simulink model "EV_Modeling_old"  (R2024b)
settings: Solver=FixedStepAuto  StartTime=0.0  StopTime=10382  FixedStep=0.1  RelTol=1e-3
values from neighbouring files (symbols this model uses):
  battery_SOC_SOC = battery_SOC(:,1)    [EV_Truck.m]    (also in simulink.m)
  battery_SOC_voltage = battery_SOC(:,2)    [EV_Truck.m]    (also in simulink.m)
  drag_coefficient_FV1 = table2array(drag_coefficient(:,3))    [simulink.m]
  drag_coefficient_FV2 = table2array(drag_coefficient(:,4))    [simulink.m]
  drag_coefficient_input = table2array(drag_coefficient(:,1))    [simulink.m]
  drag_coefficient_LV = table2array(drag_coefficient(:,2))    [simulink.m]
  electric_consumption_ressistancce = electric_consumption(:,2)    [EV_Truck.m]    (also in simulink.m)
  electric_consumption_voltage = electric_consumption(:,1)    [EV_Truck.m]    (also in simulink.m)
  motor_efficiency_efficiency = table2array(motor_efficiency(2:height(motor_efficiency),2:width(motor_efficiency)))    [EV_Truck.m]    (also in simulink.m)
  motor_efficiency_RPM = table2array(motor_efficiency(2:height(motor_efficiency),1))    [EV_Truck.m]    (also in simulink.m)
  motor_efficiency_torque = transpose(motor_efficiency_torque)    [EV_Truck.m]    (also in simulink.m)
  motor_RPM_torque = table2array(motor_torque(1:14,1))    [EV_Truck.m]    (also in simulink.m)
  motor_torque_RPM = table2array(motor_torque(1:14,2))    [EV_Truck.m]    (also in simulink.m)
undefined symbols (not defined in the file or in its folder): battery_builder_rtmsupport, battery_sli_rtmsupport, C1_mat, C2_mat, c_sqrt, DiscIntNeverNeededParam, dV0_mat, gcbh, n, Wc, Wm, x0
libraries: simulink x87, packLibrary_lib x30, nesl_utility x6, fl_lib x6, simulink_extras x3, mpcadaslib x2, slpidlib x1
(part 12 of 12)

== system EV_Modeling_old/FV2/SOC Estimator (Kalman Filter)1/Kalman Filter/UKBF 2RC/Prediction-correction/Xdot/Sigma points derivatives ==
  A : Inport
  Fi : Inport  Port=2
  x1 : Inport  Port=3
  Assignment : Assignment  NumberOfDimensions=2  DiagnosticForDimensions=Warning  IndexOptions=Index vector (dialog),Index vector (dialog)  Indices=1:n,1  OutputSizes=1,1
  Assignment1 : Assignment  NumberOfDimensions=2  DiagnosticForDimensions=Warning  IndexOptions=Index vector (dialog),Index vector (dialog)  Indices=1:n,2:n+1  OutputSizes=1,1
  Assignment2 : Assignment  NumberOfDimensions=2  DiagnosticForDimensions=Warning  IndexOptions=Index vector (dialog),Index vector (dialog)  Indices=1:n,n+2:2*n+1  OutputSizes=1,1
  Constant : Constant  Value=zeros(n,2*n+1)
  Constant1 : Constant  Value=ones(1,n)  VectorParams1D=off
  Gain : Gain  Gain=c_sqrt
  Matrix Multiply : Product  Multiplication=Matrix(*)
  Matrix Multiply1 : Product  Multiplication=Matrix(*)
  Sum : Sum  Inputs=|++
  Sum1 : Sum  Inputs=|+-
  Xdot : Outport
  wires:
  x1/1 -> Matrix Multiply/1, Assignment/2
  Constant1/1 -> Matrix Multiply/2
  Matrix Multiply/1 -> Sum1/1, Sum/1
  Gain/1 -> Sum1/2, Sum/2
  Sum/1 -> Assignment1/2
  Sum1/1 -> Assignment2/2
  Constant/1 -> Assignment/1
  Assignment/1 -> Assignment1/1
  Assignment1/1 -> Assignment2/1
  Assignment2/1 -> Xdot/1
  A/1 -> Matrix Multiply1/1
  Fi/1 -> Matrix Multiply1/2
  Matrix Multiply1/1 -> Gain/1

== system EV_Modeling_old/FV2/SOC Estimator (Kalman Filter)1/Kalman Filter/UKBF 2RC/Prediction-correction/Xdot/Update Fi ==
  A : Inport
  XWf : Inport  Port=2
  fWX : Inport  Port=3
  K : Inport  Port=4
  Constant1 : Constant  Value=double(Q_2RC)
  Constant4 : Constant  Value=eye(size(P0_2RC,1))
  Constant5 : Constant  Value=double(R)
  Divide1 : Product  Inputs=*/  Multiplication=Matrix(*)
  Gain5 : Gain  Gain=tril(ones(n)-diag(0.5*ones(1,n)))
  Matrix Multiply7 : Product  Inputs=3  Multiplication=Matrix(*)
  Matrix Multiply8 : Product  Inputs=3  Multiplication=Matrix(*)
  Sum3 : Sum  Inputs=+++-
  Transpose3 : Math  Operator=transpose
  Transpose4 : Math  Operator=transpose
  Fi : Outport
  wires:
  A/1 -> Divide1/2
  Matrix Multiply7/1 -> Gain5/1  "M"
  Constant1/1 -> Sum3/3
  Sum3/1 -> Matrix Multiply7/2
  Transpose3/1 -> Matrix Multiply8/3
  Matrix Multiply8/1 -> Sum3/4
  Divide1/1 -> Transpose4/1, Matrix Multiply7/1
  K/1 -> Transpose3/1, Matrix Multiply8/1
  XWf/1 -> Sum3/1
  Constant4/1 -> Divide1/1
  Transpose4/1 -> Matrix Multiply7/3
  Constant5/1 -> Matrix Multiply8/2
  fWX/1 -> Sum3/2
  Gain5/1 -> Fi/1  "Fi"

== system EV_Modeling_old/FV2/SOC Estimator (Kalman Filter)1/Kalman Filter/UKF/Prediction/Measurement function/Measurement function ==
  Current : Inport
  Temperature : Inport  Port=2
  x : Inport  Port=3
  Add2 : Sum  Inputs=+--
  Get SOC : Selector  InputPortWidth=2  IndexOptions=Index vector (dialog)  Indices=[1]  OutputSizes=1
  Get V1 : Selector  InputPortWidth=2  IndexOptions=Index vector (dialog)  Indices=2  OutputSizes=1
  OCV Table : Lookup_n-D  BreakpointsForDimension1=SOC_vec  BreakpointsForDimension2=T_vec  BeginIndexSearchUsingPreviousIndexResult=on  Table=V0_mat  ExtrapMethod=Clip  InternalRulePriority=Speed  RndMeth=Simplest
      settings: InputPortMap=u0,u1
  Product2 : Product
  R0 Table : Lookup_n-D  BreakpointsForDimension1=SOC_vec  BreakpointsForDimension2=T_vec  BeginIndexSearchUsingPreviousIndexResult=on  Table=R0_mat  ExtrapMethod=Clip  InternalRulePriority=Speed  RndMeth=Simplest
      settings: InputPortMap=u0,u1
  y : Outport
  wires:
  x/1 -> Get SOC/1, Get V1/1
  OCV Table/1 -> Add2/1
  Current/1 -> Product2/2
  Get SOC/1 -> OCV Table/1, R0 Table/1
  Get V1/1 -> Add2/3  "U1"
  Product2/1 -> Add2/2
  Add2/1 -> y/1
  R0 Table/1 -> Product2/1
  Temperature/1 -> R0 Table/2, OCV Table/2

== system EV_Modeling_old/FV2/SOC Estimator (Kalman Filter)1/Kalman Filter/UKF/Prediction/State function/State function ==
  Current : Inport
  Temperature : Inport  Port=2
  x : Inport  Port=3
  Add : Sum
  Add1 : Sum  Inputs=-+
  C1 : Lookup_n-D  BreakpointsForDimension1=SOC_vec  BreakpointsForDimension2=T_vec  BeginIndexSearchUsingPreviousIndexResult=on  Table=C1_mat  ExtrapMethod=Clip  InternalRulePriority=Speed  RndMeth=Simplest
      settings: InputPortMap=u0,u1
  Divide1 : Product  Inputs=*/
  Divide2 : Product  Inputs=*/
  Gain : Gain  Gain=-1/(AH*3600)
  Get SOC : Selector  InputPortWidth=2  IndexOptions=Index vector (dialog)  Indices=1  OutputSizes=1
  Get V1 : Selector  InputPortWidth=2  IndexOptions=Index vector (dialog)  Indices=2  OutputSizes=1
  Mux : Mux  Inputs=2
  Probe : Probe  ProbeWidth=off  ProbeComplexSignal=off  ProbeSampleTimeDataType=Same as input
  Product : Product  OutDataTypeStr=single
  Product1 : Product
  R1 : Lookup_n-D  BreakpointsForDimension1=SOC_vec  BreakpointsForDimension2=T_vec  BeginIndexSearchUsingPreviousIndexResult=on  Table=R1_mat  ExtrapMethod=Clip  InternalRulePriority=Speed  RndMeth=Simplest
      settings: InputPortMap=u0,u1
  Selector : Selector  InputPortWidth=2  IndexOptions=Index vector (dialog)  Indices=1  OutputSizes=1
  xk1 : Outport
  wires:
  Gain/1 -> Mux/1
  Temperature/1 -> R1/2, C1/2
  x/1 -> Get SOC/1, Get V1/1, Add/1
  Product/1 -> Add/2
  Add1/1 -> Mux/2  "xdot_2"
  Add/1 -> xk1/1
  Divide2/1 -> Add1/1
  Mux/1 -> Product/1  "xdot"
  Selector/1 -> Product/2
  Current/1 -> Probe/1, Divide1/1, Gain/1  "Current"
  C1/1 -> Divide1/2, Product1/2  "C1"
  Get V1/1 -> Divide2/1
  R1/1 -> Product1/1  "R1"
  Get SOC/1 -> R1/1, C1/1
  Product1/1 -> Divide2/2  "R1*C1"
  Divide1/1 -> Add1/2  "Current/C1"
  Probe/1 -> Selector/1

== system EV_Modeling_old/FV2/SOC Estimator (Kalman Filter)1/Kalman Filter/UKF 2RC/Prediction/Measurement function/Measurement function ==
  Current : Inport
  Temperature : Inport  Port=2
  x : Inport  Port=3
  Add2 : Sum  Inputs=+---
  Get SOC : Selector  InputPortWidth=3  IndexOptions=Index vector (dialog)  Indices=[1]  OutputSizes=1
  Get V1 : Selector  InputPortWidth=3  IndexOptions=Index vector (dialog)  Indices=2  OutputSizes=1
  Get V2 : Selector  InputPortWidth=3  IndexOptions=Index vector (dialog)  Indices=3  OutputSizes=1
  OCV Table : Lookup_n-D  BreakpointsForDimension1=SOC_vec  BreakpointsForDimension2=T_vec  BeginIndexSearchUsingPreviousIndexResult=on  Table=V0_mat  ExtrapMethod=Clip  InternalRulePriority=Speed  RndMeth=Simplest
      settings: InputPortMap=u0,u1
  Product2 : Product
  R0 Table : Lookup_n-D  BreakpointsForDimension1=SOC_vec  BreakpointsForDimension2=T_vec  BeginIndexSearchUsingPreviousIndexResult=on  Table=R0_mat  ExtrapMethod=Clip  InternalRulePriority=Speed  RndMeth=Simplest
      settings: InputPortMap=u0,u1
  y : Outport
  wires:
  Get V2/1 -> Add2/4  "V2"
  x/1 -> Get SOC/1, Get V1/1, Get V2/1
  OCV Table/1 -> Add2/1
  Current/1 -> Product2/2
  Get SOC/1 -> OCV Table/1, R0 Table/1
  Get V1/1 -> Add2/3  "V1"
  Product2/1 -> Add2/2
  Add2/1 -> y/1
  R0 Table/1 -> Product2/1
  Temperature/1 -> R0 Table/2, OCV Table/2

== system EV_Modeling_old/FV2/SOC Estimator (Kalman Filter)1/Kalman Filter/UKF 2RC/Prediction/State function/State function ==
  Current : Inport
  Temperature : Inport  Port=2
  x : Inport  Port=3
  Add : Sum
  Add1 : Sum  Inputs=-+
  Add2 : Sum  Inputs=-+
  C1 : Lookup_n-D  BreakpointsForDimension1=SOC_vec  BreakpointsForDimension2=T_vec  BeginIndexSearchUsingPreviousIndexResult=on  Table=C1_mat  ExtrapMethod=Clip  InternalRulePriority=Speed  RndMeth=Simplest
      settings: InputPortMap=u0,u1
  C2 : Lookup_n-D  BreakpointsForDimension1=SOC_vec  BreakpointsForDimension2=T_vec  Table=C2_mat  InternalRulePriority=Speed  RndMeth=Simplest
      settings: InputPortMap=u0,u1
  Divide{1..4} (4 alike) : Product  Inputs=*/
  Gain : Gain  Gain=-1/(AH*3600)
  Get SOC : Selector  InputPortWidth=3  IndexOptions=Index vector (dialog)  Indices=1  OutputSizes=1
  Get V1 : Selector  InputPortWidth=3  IndexOptions=Index vector (dialog)  Indices=2  OutputSizes=1
  Get V2 : Selector  InputPortWidth=3  IndexOptions=Index vector (dialog)  Indices=3  OutputSizes=1
  Mux : Mux  Inputs=3
  Probe : Probe  ProbeWidth=off  ProbeComplexSignal=off  ProbeSampleTimeDataType=Same as input
  Product : Product  OutDataTypeStr=single
  Product1 : Product
  Product2 : Product
  R1 : Lookup_n-D  BreakpointsForDimension1=SOC_vec  BreakpointsForDimension2=T_vec  BeginIndexSearchUsingPreviousIndexResult=on  Table=R1_mat  ExtrapMethod=Clip  InternalRulePriority=Speed  RndMeth=Simplest
      settings: InputPortMap=u0,u1
  R2 : Lookup_n-D  BreakpointsForDimension1=SOC_vec  BreakpointsForDimension2=T_vec  Table=R2_mat  InternalRulePriority=Speed  RndMeth=Simplest
      settings: InputPortMap=u0,u1
  Selector : Selector  InputPortWidth=2  IndexOptions=Index vector (dialog)  Indices=1  OutputSizes=1
  xk1 : Outport
  wires:
  Get V2/1 -> Divide3/1
  Add2/1 -> Mux/3  "xdot_3"
  Divide4/1 -> Add2/2  "Current/C2"
  Divide3/1 -> Add2/1
  Product2/1 -> Divide3/2  "R2*C2"
  C2/1 -> Product2/2, Divide4/2  "C2"
  R2/1 -> Product2/1  "R2"
  Gain/1 -> Mux/1
  Temperature/1 -> R1/2, C1/2, R2/2, C2/2
  x/1 -> Get SOC/1, Get V1/1, Add/1, Get V2/1
  Product/1 -> Add/2
  Add1/1 -> Mux/2  "xdot_2"
  Add/1 -> xk1/1
  Divide2/1 -> Add1/1
  Mux/1 -> Product/1  "xdot"
  Selector/1 -> Product/2
  Current/1 -> Probe/1, Divide1/1, Gain/1, Divide4/1  "Current"
  C1/1 -> Divide1/2, Product1/2  "C1"
  Get V1/1 -> Divide2/1
  R1/1 -> Product1/1  "R1"
  Get SOC/1 -> R1/1, C1/1, R2/1, C2/1
  Product1/1 -> Divide2/2  "R1*C1"
  Divide1/1 -> Add1/2  "Current/C1"
  Probe/1 -> Selector/1

== system EV_Modeling_old/LV/SOC Estimator (Kalman Filter)/Kalman Filter/UKBF/Prediction-correction/Measurement function/Measurement function ==
  Current : Inport
  Temperature : Inport  Port=2
  x : Inport  Port=3
  Add2 : Sum  Inputs=+--
  Get SOC1 : Selector  InputPortWidth=2  IndexOptions=Index vector (dialog)  Indices=[1]  OutputSizes=1
  Get V1 : Selector  InputPortWidth=2  IndexOptions=Index vector (dialog)  Indices=2  OutputSizes=1
  OCV Table : Lookup_n-D  BreakpointsForDimension1=SOC_vec  BreakpointsForDimension2=T_vec  BeginIndexSearchUsingPreviousIndexResult=on  Table=V0_mat  ExtrapMethod=Clip  InternalRulePriority=Speed  RndMeth=Simplest
      settings: InputPortMap=u0,u1
  Product2 : Product
  R0 Table : Lookup_n-D  BreakpointsForDimension1=SOC_vec  BreakpointsForDimension2=T_vec  BeginIndexSearchUsingPreviousIndexResult=on  Table=R0_mat  ExtrapMethod=Clip  InternalRulePriority=Speed  RndMeth=Simplest
      settings: InputPortMap=u0,u1
  y : Outport
  wires:
  x/1 -> Get SOC1/1, Get V1/1
  OCV Table/1 -> Add2/1
  Current/1 -> Product2/2
  Get SOC1/1 -> OCV Table/1, R0 Table/1  "SOC"
  Get V1/1 -> Add2/3
  Product2/1 -> Add2/2
  Add2/1 -> y/1
  R0 Table/1 -> Product2/1
  Temperature/1 -> R0 Table/2, OCV Table/2

== system EV_Modeling_old/LV/SOC Estimator (Kalman Filter)/Kalman Filter/UKBF/Prediction-correction/State function/State function ==
  Current : Inport
  Temperature : Inport  Port=2
  x : Inport  Port=3
  Add1 : Sum  Inputs=-+
  C1 : Lookup_n-D  BreakpointsForDimension1=SOC_vec  BreakpointsForDimension2=T_vec  BeginIndexSearchUsingPreviousIndexResult=on  Table=C1_mat  ExtrapMethod=Clip  InternalRulePriority=Speed  RndMeth=Simplest
      settings: InputPortMap=u0,u1
  Divide1 : Product  Inputs=*/
  Divide2 : Product  Inputs=*/
  Gain : Gain  Gain=-1/(AH*3600)
  Get SOC : Selector  InputPortWidth=2  IndexOptions=Index vector (dialog)  Indices=1  OutputSizes=1
  Get V1 : Selector  InputPortWidth=2  IndexOptions=Index vector (dialog)  Indices=2  OutputSizes=1
  Mux : Mux  Inputs=2
  Product1 : Product
  R1 : Lookup_n-D  BreakpointsForDimension1=SOC_vec  BreakpointsForDimension2=T_vec  BeginIndexSearchUsingPreviousIndexResult=on  Table=R1_mat  ExtrapMethod=Clip  InternalRulePriority=Speed  RndMeth=Simplest
      settings: InputPortMap=u0,u1
  f(x) : Outport
  wires:
  Gain/1 -> Mux/1
  Temperature/1 -> R1/2, C1/2
  x/1 -> Get SOC/1, Get V1/1
  Add1/1 -> Mux/2  "xdot_2"
  Divide2/1 -> Add1/1
  Mux/1 -> f(x)/1  "xdot"
  Current/1 -> Divide1/1, Gain/1  "Current"
  C1/1 -> Divide1/2, Product1/2  "C1"
  Get V1/1 -> Divide2/1  "V1"
  R1/1 -> Product1/1  "R1"
  Get SOC/1 -> R1/1, C1/1
  Product1/1 -> Divide2/2  "R1*C1"
  Divide1/1 -> Add1/2  "Current/C1"

== system EV_Modeling_old/LV/SOC Estimator (Kalman Filter)/Kalman Filter/UKBF/Prediction-correction/Xdot/Sigma points derivatives ==
  A : Inport
  Fi : Inport  Port=2
  x1 : Inport  Port=3
  Assignment : Assignment  NumberOfDimensions=2  DiagnosticForDimensions=Warning  IndexOptions=Index vector (dialog),Index vector (dialog)  Indices=1:n,1  OutputSizes=1,1
  Assignment1 : Assignment  NumberOfDimensions=2  DiagnosticForDimensions=Warning  IndexOptions=Index vector (dialog),Index vector (dialog)  Indices=1:n,2:n+1  OutputSizes=1,1
  Assignment2 : Assignment  NumberOfDimensions=2  DiagnosticForDimensions=Warning  IndexOptions=Index vector (dialog),Index vector (dialog)  Indices=1:n,n+2:2*n+1  OutputSizes=1,1
  Constant : Constant  Value=zeros(n,2*n+1)
  Constant1 : Constant  Value=ones(1,n)  VectorParams1D=off
  Gain : Gain  Gain=c_sqrt
  Matrix Multiply : Product  Multiplication=Matrix(*)
  Matrix Multiply1 : Product  Multiplication=Matrix(*)
  Sum : Sum  Inputs=|++
  Sum1 : Sum  Inputs=|+-
  Xdot : Outport
  wires:
  x1/1 -> Matrix Multiply/1, Assignment/2
  Constant1/1 -> Matrix Multiply/2
  Matrix Multiply/1 -> Sum1/1, Sum/1
  Gain/1 -> Sum1/2, Sum/2
  Sum/1 -> Assignment1/2
  Sum1/1 -> Assignment2/2
  Constant/1 -> Assignment/1
  Assignment/1 -> Assignment1/1
  Assignment1/1 -> Assignment2/1
  Assignment2/1 -> Xdot/1
  A/1 -> Matrix Multiply1/1
  Fi/1 -> Matrix Multiply1/2
  Matrix Multiply1/1 -> Gain/1

== system EV_Modeling_old/LV/SOC Estimator (Kalman Filter)/Kalman Filter/UKBF/Prediction-correction/Xdot/Update Fi ==
  A : Inport
  XWf : Inport  Port=2
  fWX : Inport  Port=3
  K : Inport  Port=4
  Constant1 : Constant  Value=double(Q)
  Constant4 : Constant  Value=eye(size(P0,1))
  Constant5 : Constant  Value=double(R)
  Divide1 : Product  Inputs=*/  Multiplication=Matrix(*)
  Gain5 : Gain  Gain=tril(ones(n)-diag(0.5*ones(1,n)))
  Matrix Multiply7 : Product  Inputs=3  Multiplication=Matrix(*)
  Matrix Multiply8 : Product  Inputs=3  Multiplication=Matrix(*)
  Sum3 : Sum  Inputs=+++-
  Transpose3 : Math  Operator=transpose
  Transpose4 : Math  Operator=transpose
  Fi : Outport
  wires:
  A/1 -> Divide1/2
  Matrix Multiply7/1 -> Gain5/1  "M"
  Constant1/1 -> Sum3/3
  Sum3/1 -> Matrix Multiply7/2
  Transpose3/1 -> Matrix Multiply8/3
  Matrix Multiply8/1 -> Sum3/4
  Divide1/1 -> Transpose4/1, Matrix Multiply7/1
  K/1 -> Transpose3/1, Matrix Multiply8/1
  XWf/1 -> Sum3/1
  Constant4/1 -> Divide1/1
  Transpose4/1 -> Matrix Multiply7/3
  Constant5/1 -> Matrix Multiply8/2
  fWX/1 -> Sum3/2
  Gain5/1 -> Fi/1  "Fi"

== system EV_Modeling_old/LV/SOC Estimator (Kalman Filter)/Kalman Filter/UKBF 2RC/Prediction-correction/Measurement function/Measurement function ==
  Current : Inport
  Temperature : Inport  Port=2
  x : Inport  Port=3
  Add2 : Sum  Inputs=+---
  Get SOC1 : Selector  InputPortWidth=3  IndexOptions=Index vector (dialog)  Indices=[1]  OutputSizes=1
  Get V1 : Selector  InputPortWidth=3  IndexOptions=Index vector (dialog)  Indices=2  OutputSizes=1
  Get V2 : Selector  InputPortWidth=3  IndexOptions=Index vector (dialog)  Indices=3  OutputSizes=1
  OCV Table : Lookup_n-D  BreakpointsForDimension1=SOC_vec  BreakpointsForDimension2=T_vec  BeginIndexSearchUsingPreviousIndexResult=on  Table=V0_mat  ExtrapMethod=Clip  InternalRulePriority=Speed  RndMeth=Simplest
      settings: InputPortMap=u0,u1
  Product2 : Product
  R0 Table : Lookup_n-D  BreakpointsForDimension1=SOC_vec  BreakpointsForDimension2=T_vec  BeginIndexSearchUsingPreviousIndexResult=on  Table=R0_mat  ExtrapMethod=Clip  InternalRulePriority=Speed  RndMeth=Simplest
      settings: InputPortMap=u0,u1
  y : Outport
  wires:
  Get V2/1 -> Add2/4
  x/1 -> Get SOC1/1, Get V1/1, Get V2/1
  OCV Table/1 -> Add2/1
  Current/1 -> Product2/2
  Get SOC1/1 -> OCV Table/1, R0 Table/1  "SOC"
  Get V1/1 -> Add2/3
  Product2/1 -> Add2/2
  Add2/1 -> y/1
  R0 Table/1 -> Product2/1
  Temperature/1 -> R0 Table/2, OCV Table/2

== system EV_Modeling_old/LV/SOC Estimator (Kalman Filter)/Kalman Filter/UKBF 2RC/Prediction-correction/State function/State function ==
  Current : Inport
  Temperature : Inport  Port=2
  x : Inport  Port=3
  2-D Lookup Table C2 : Lookup_n-D  BreakpointsForDimension1=SOC_vec  BreakpointsForDimension2=T_vec  Table=C2_mat  InternalRulePriority=Speed  RndMeth=Simplest
      settings: InputPortMap=u0,u1
  2-D Lookup Table R2 : Lookup_n-D  BreakpointsForDimension1=SOC_vec  BreakpointsForDimension2=T_vec  Table=R2_mat  InternalRulePriority=Speed  RndMeth=Simplest
      settings: InputPortMap=u0,u1
  Add1 : Sum  Inputs=-+
  Add2 : Sum  Inputs=-+
  C1 : Lookup_n-D  BreakpointsForDimension1=SOC_vec  BreakpointsForDimension2=T_vec  BeginIndexSearchUsingPreviousIndexResult=on  Table=C1_mat  ExtrapMethod=Clip  InternalRulePriority=Speed  RndMeth=Simplest
      settings: InputPortMap=u0,u1
  Divide{1..4} (4 alike) : Product  Inputs=*/
  Gain : Gain  Gain=-1/(AH*3600)
  Get SOC : Selector  InputPortWidth=3  IndexOptions=Index vector (dialog)  Indices=1  OutputSizes=1
  Get V1 : Selector  InputPortWidth=3  IndexOptions=Index vector (dialog)  Indices=2  OutputSizes=1
  Get V2 : Selector  InputPortWidth=3  IndexOptions=Index vector (dialog)  Indices=3  OutputSizes=1
  Mux : Mux  Inputs=3
  Product1 : Product
  Product2 : Product
  R1 : Lookup_n-D  BreakpointsForDimension1=SOC_vec  BreakpointsForDimension2=T_vec  BeginIndexSearchUsingPreviousIndexResult=on  Table=R1_mat  ExtrapMethod=Clip  InternalRulePriority=Speed  RndMeth=Simplest
      settings: InputPortMap=u0,u1
  f(x) : Outport
  wires:
  Divide4/1 -> Add2/2  "Current/C2"
  Divide3/1 -> Add2/1
  Add2/1 -> Mux/3  "xdot_3"
  Product2/1 -> Divide3/2  "R1*C1"
  Get V2/1 -> Divide3/1  "V2"
  2-D Lookup Table C2/1 -> Product2/2, Divide4/2  "C2"
  2-D Lookup Table R2/1 -> Product2/1  "R2"
  Gain/1 -> Mux/1
  Temperature/1 -> R1/2, C1/2, 2-D Lookup Table R2/2, 2-D Lookup Table C2/2
  x/1 -> Get SOC/1, Get V1/1, Get V2/1
  Add1/1 -> Mux/2  "xdot_2"
  Divide2/1 -> Add1/1
  Mux/1 -> f(x)/1  "xdot"
  Current/1 -> Divide1/1, Gain/1, Divide4/1  "Current"
  C1/1 -> Divide1/2, Product1/2  "C1"
  Get V1/1 -> Divide2/1  "V1"
  R1/1 -> Product1/1  "R1"
  Get SOC/1 -> R1/1, C1/1, 2-D Lookup Table R2/1, 2-D Lookup Table C2/1
  Product1/1 -> Divide2/2  "R1*C1"
  Divide1/1 -> Add1/2  "Current/C1"

== system EV_Modeling_old/LV/SOC Estimator (Kalman Filter)/Kalman Filter/UKBF 2RC/Prediction-correction/Xdot/Sigma points derivatives ==
  A : Inport
  Fi : Inport  Port=2
  x1 : Inport  Port=3
  Assignment : Assignment  NumberOfDimensions=2  DiagnosticForDimensions=Warning  IndexOptions=Index vector (dialog),Index vector (dialog)  Indices=1:n,1  OutputSizes=1,1
  Assignment1 : Assignment  NumberOfDimensions=2  DiagnosticForDimensions=Warning  IndexOptions=Index vector (dialog),Index vector (dialog)  Indices=1:n,2:n+1  OutputSizes=1,1
  Assignment2 : Assignment  NumberOfDimensions=2  DiagnosticForDimensions=Warning  IndexOptions=Index vector (dialog),Index vector (dialog)  Indices=1:n,n+2:2*n+1  OutputSizes=1,1
  Constant : Constant  Value=zeros(n,2*n+1)
  Constant1 : Constant  Value=ones(1,n)  VectorParams1D=off
  Gain : Gain  Gain=c_sqrt
  Matrix Multiply : Product  Multiplication=Matrix(*)
  Matrix Multiply1 : Product  Multiplication=Matrix(*)
  Sum : Sum  Inputs=|++
  Sum1 : Sum  Inputs=|+-
  Xdot : Outport
  wires:
  x1/1 -> Matrix Multiply/1, Assignment/2
  Constant1/1 -> Matrix Multiply/2
  Matrix Multiply/1 -> Sum1/1, Sum/1
  Gain/1 -> Sum1/2, Sum/2
  Sum/1 -> Assignment1/2
  Sum1/1 -> Assignment2/2
  Constant/1 -> Assignment/1
  Assignment/1 -> Assignment1/1
  Assignment1/1 -> Assignment2/1
  Assignment2/1 -> Xdot/1
  A/1 -> Matrix Multiply1/1
  Fi/1 -> Matrix Multiply1/2
  Matrix Multiply1/1 -> Gain/1

== system EV_Modeling_old/LV/SOC Estimator (Kalman Filter)/Kalman Filter/UKBF 2RC/Prediction-correction/Xdot/Update Fi ==
  A : Inport
  XWf : Inport  Port=2
  fWX : Inport  Port=3
  K : Inport  Port=4
  Constant1 : Constant  Value=double(Q_2RC)
  Constant4 : Constant  Value=eye(size(P0_2RC,1))
  Constant5 : Constant  Value=double(R)
  Divide1 : Product  Inputs=*/  Multiplication=Matrix(*)
  Gain5 : Gain  Gain=tril(ones(n)-diag(0.5*ones(1,n)))
  Matrix Multiply7 : Product  Inputs=3  Multiplication=Matrix(*)
  Matrix Multiply8 : Product  Inputs=3  Multiplication=Matrix(*)
  Sum3 : Sum  Inputs=+++-
  Transpose3 : Math  Operator=transpose
  Transpose4 : Math  Operator=transpose
  Fi : Outport
  wires:
  A/1 -> Divide1/2
  Matrix Multiply7/1 -> Gain5/1  "M"
  Constant1/1 -> Sum3/3
  Sum3/1 -> Matrix Multiply7/2
  Transpose3/1 -> Matrix Multiply8/3
  Matrix Multiply8/1 -> Sum3/4
  Divide1/1 -> Transpose4/1, Matrix Multiply7/1
  K/1 -> Transpose3/1, Matrix Multiply8/1
  XWf/1 -> Sum3/1
  Constant4/1 -> Divide1/1
  Transpose4/1 -> Matrix Multiply7/3
  Constant5/1 -> Matrix Multiply8/2
  fWX/1 -> Sum3/2
  Gain5/1 -> Fi/1  "Fi"

== system EV_Modeling_old/LV/SOC Estimator (Kalman Filter)/Kalman Filter/UKF/Prediction/Measurement function/Measurement function ==
  Current : Inport
  Temperature : Inport  Port=2
  x : Inport  Port=3
  Add2 : Sum  Inputs=+--
  Get SOC : Selector  InputPortWidth=2  IndexOptions=Index vector (dialog)  Indices=[1]  OutputSizes=1
  Get V1 : Selector  InputPortWidth=2  IndexOptions=Index vector (dialog)  Indices=2  OutputSizes=1
  OCV Table : Lookup_n-D  BreakpointsForDimension1=SOC_vec  BreakpointsForDimension2=T_vec  BeginIndexSearchUsingPreviousIndexResult=on  Table=V0_mat  ExtrapMethod=Clip  InternalRulePriority=Speed  RndMeth=Simplest
      settings: InputPortMap=u0,u1
  Product2 : Product
  R0 Table : Lookup_n-D  BreakpointsForDimension1=SOC_vec  BreakpointsForDimension2=T_vec  BeginIndexSearchUsingPreviousIndexResult=on  Table=R0_mat  ExtrapMethod=Clip  InternalRulePriority=Speed  RndMeth=Simplest
      settings: InputPortMap=u0,u1
  y : Outport
  wires:
  x/1 -> Get SOC/1, Get V1/1
  OCV Table/1 -> Add2/1
  Current/1 -> Product2/2
  Get SOC/1 -> OCV Table/1, R0 Table/1
  Get V1/1 -> Add2/3  "U1"
  Product2/1 -> Add2/2
  Add2/1 -> y/1
  R0 Table/1 -> Product2/1
  Temperature/1 -> R0 Table/2, OCV Table/2

== system EV_Modeling_old/LV/SOC Estimator (Kalman Filter)/Kalman Filter/UKF/Prediction/State function/State function ==
  Current : Inport
  Temperature : Inport  Port=2
  x : Inport  Port=3
  Add : Sum
  Add1 : Sum  Inputs=-+
  C1 : Lookup_n-D  BreakpointsForDimension1=SOC_vec  BreakpointsForDimension2=T_vec  BeginIndexSearchUsingPreviousIndexResult=on  Table=C1_mat  ExtrapMethod=Clip  InternalRulePriority=Speed  RndMeth=Simplest
      settings: InputPortMap=u0,u1
  Divide1 : Product  Inputs=*/
  Divide2 : Product  Inputs=*/
  Gain : Gain  Gain=-1/(AH*3600)
  Get SOC : Selector  InputPortWidth=2  IndexOptions=Index vector (dialog)  Indices=1  OutputSizes=1
  Get V1 : Selector  InputPortWidth=2  IndexOptions=Index vector (dialog)  Indices=2  OutputSizes=1
  Mux : Mux  Inputs=2
  Probe : Probe  ProbeWidth=off  ProbeComplexSignal=off  ProbeSampleTimeDataType=Same as input
  Product : Product  OutDataTypeStr=single
  Product1 : Product
  R1 : Lookup_n-D  BreakpointsForDimension1=SOC_vec  BreakpointsForDimension2=T_vec  BeginIndexSearchUsingPreviousIndexResult=on  Table=R1_mat  ExtrapMethod=Clip  InternalRulePriority=Speed  RndMeth=Simplest
      settings: InputPortMap=u0,u1
  Selector : Selector  InputPortWidth=2  IndexOptions=Index vector (dialog)  Indices=1  OutputSizes=1
  xk1 : Outport
  wires:
  Gain/1 -> Mux/1
  Temperature/1 -> R1/2, C1/2
  x/1 -> Get SOC/1, Get V1/1, Add/1
  Product/1 -> Add/2
  Add1/1 -> Mux/2  "xdot_2"
  Add/1 -> xk1/1
  Divide2/1 -> Add1/1
  Mux/1 -> Product/1  "xdot"
  Selector/1 -> Product/2
  Current/1 -> Probe/1, Divide1/1, Gain/1  "Current"
  C1/1 -> Divide1/2, Product1/2  "C1"
  Get V1/1 -> Divide2/1
  R1/1 -> Product1/1  "R1"
  Get SOC/1 -> R1/1, C1/1
  Product1/1 -> Divide2/2  "R1*C1"
  Divide1/1 -> Add1/2  "Current/C1"
  Probe/1 -> Selector/1

== system EV_Modeling_old/LV/SOC Estimator (Kalman Filter)/Kalman Filter/UKF 2RC/Prediction/Measurement function/Measurement function ==
  Current : Inport
  Temperature : Inport  Port=2
  x : Inport  Port=3
  Add2 : Sum  Inputs=+---
  Get SOC : Selector  InputPortWidth=3  IndexOptions=Index vector (dialog)  Indices=[1]  OutputSizes=1
  Get V1 : Selector  InputPortWidth=3  IndexOptions=Index vector (dialog)  Indices=2  OutputSizes=1
  Get V2 : Selector  InputPortWidth=3  IndexOptions=Index vector (dialog)  Indices=3  OutputSizes=1
  OCV Table : Lookup_n-D  BreakpointsForDimension1=SOC_vec  BreakpointsForDimension2=T_vec  BeginIndexSearchUsingPreviousIndexResult=on  Table=V0_mat  ExtrapMethod=Clip  InternalRulePriority=Speed  RndMeth=Simplest
      settings: InputPortMap=u0,u1
  Product2 : Product
  R0 Table : Lookup_n-D  BreakpointsForDimension1=SOC_vec  BreakpointsForDimension2=T_vec  BeginIndexSearchUsingPreviousIndexResult=on  Table=R0_mat  ExtrapMethod=Clip  InternalRulePriority=Speed  RndMeth=Simplest
      settings: InputPortMap=u0,u1
  y : Outport
  wires:
  Get V2/1 -> Add2/4  "V2"
  x/1 -> Get SOC/1, Get V1/1, Get V2/1
  OCV Table/1 -> Add2/1
  Current/1 -> Product2/2
  Get SOC/1 -> OCV Table/1, R0 Table/1
  Get V1/1 -> Add2/3  "V1"
  Product2/1 -> Add2/2
  Add2/1 -> y/1
  R0 Table/1 -> Product2/1
  Temperature/1 -> R0 Table/2, OCV Table/2

== system EV_Modeling_old/LV/SOC Estimator (Kalman Filter)/Kalman Filter/UKF 2RC/Prediction/State function/State function ==
  Current : Inport
  Temperature : Inport  Port=2
  x : Inport  Port=3
  Add : Sum
  Add1 : Sum  Inputs=-+
  Add2 : Sum  Inputs=-+
  C1 : Lookup_n-D  BreakpointsForDimension1=SOC_vec  BreakpointsForDimension2=T_vec  BeginIndexSearchUsingPreviousIndexResult=on  Table=C1_mat  ExtrapMethod=Clip  InternalRulePriority=Speed  RndMeth=Simplest
      settings: InputPortMap=u0,u1
  C2 : Lookup_n-D  BreakpointsForDimension1=SOC_vec  BreakpointsForDimension2=T_vec  Table=C2_mat  InternalRulePriority=Speed  RndMeth=Simplest
      settings: InputPortMap=u0,u1
  Divide{1..4} (4 alike) : Product  Inputs=*/
  Gain : Gain  Gain=-1/(AH*3600)
  Get SOC : Selector  InputPortWidth=3  IndexOptions=Index vector (dialog)  Indices=1  OutputSizes=1
  Get V1 : Selector  InputPortWidth=3  IndexOptions=Index vector (dialog)  Indices=2  OutputSizes=1
  Get V2 : Selector  InputPortWidth=3  IndexOptions=Index vector (dialog)  Indices=3  OutputSizes=1
  Mux : Mux  Inputs=3
  Probe : Probe  ProbeWidth=off  ProbeComplexSignal=off  ProbeSampleTimeDataType=Same as input
  Product : Product  OutDataTypeStr=single
  Product1 : Product
  Product2 : Product
  R1 : Lookup_n-D  BreakpointsForDimension1=SOC_vec  BreakpointsForDimension2=T_vec  BeginIndexSearchUsingPreviousIndexResult=on  Table=R1_mat  ExtrapMethod=Clip  InternalRulePriority=Speed  RndMeth=Simplest
      settings: InputPortMap=u0,u1
  R2 : Lookup_n-D  BreakpointsForDimension1=SOC_vec  BreakpointsForDimension2=T_vec  Table=R2_mat  InternalRulePriority=Speed  RndMeth=Simplest
      settings: InputPortMap=u0,u1
  Selector : Selector  InputPortWidth=2  IndexOptions=Index vector (dialog)  Indices=1  OutputSizes=1
  xk1 : Outport
  wires:
  Get V2/1 -> Divide3/1
  Add2/1 -> Mux/3  "xdot_3"
  Divide4/1 -> Add2/2  "Current/C2"
  Divide3/1 -> Add2/1
  Product2/1 -> Divide3/2  "R2*C2"
  C2/1 -> Product2/2, Divide4/2  "C2"
  R2/1 -> Product2/1  "R2"
  Gain/1 -> Mux/1
  Temperature/1 -> R1/2, C1/2, R2/2, C2/2
  x/1 -> Get SOC/1, Get V1/1, Add/1, Get V2/1
  Product/1 -> Add/2
  Add1/1 -> Mux/2  "xdot_2"
  Add/1 -> xk1/1
  Divide2/1 -> Add1/1
  Mux/1 -> Product/1  "xdot"
  Selector/1 -> Product/2
  Current/1 -> Probe/1, Divide1/1, Gain/1, Divide4/1  "Current"
  C1/1 -> Divide1/2, Product1/2  "C1"
  Get V1/1 -> Divide2/1
  R1/1 -> Product1/1  "R1"
  Get SOC/1 -> R1/1, C1/1, R2/1, C2/1
  Product1/1 -> Divide2/2  "R1*C1"
  Divide1/1 -> Add1/2  "Current/C1"
  Probe/1 -> Selector/1

== matlab function EV_Modeling_old/FV1/SOC Estimator (Kalman Filter)1/Kalman Filter/UKF 2RC/Prediction/updatePy ==
  data: Y input; y input; Py output; Y1 output; Wc parameter; R parameter
function [Py,Y1]=updatePy(Y,y, Wc, R)
% Transformed square root of covariance matrix
%Inputs:
%    Y  : Sigma points
%    y  : yhat(k+1|k)
%    Wc : Covariance weight 
%    R  : Covariance of the measurement noise
%Outputs:
%    Py: transformed square root of covariance
%    Y1: transformed deviations

[Py,Y1]=battery.control.estimators.UnscentedTransformationUpdate(Y,y, Wc, R);

== matlab function EV_Modeling_old/FV2/ACC system/MATLAB Function ==
  data: accel input; acceleration output
function acceleration  = fcn(accel)

if accel > 0 
    acceleration = (accel * 100)/0.15;
elseif accel < 0 
    acceleration = (accel * 100)/0.33;
else
    acceleration = 0; % accel이 0이거나 NaN일 경우에도 대응
end

== matlab function EV_Modeling_old/FV2/MATLAB Function ==
  data: Pmotor input; Vbatt input; R output
function R = calcResistance(Pmotor, Vbatt)
    if Pmotor == 0
        R = 1e6; % 매우 큰 저항값으로 설정 (무부하 상태 가정)
    else
        R = (Vbatt^2) / Pmotor;
    end
end

== matlab function EV_Modeling_old/FV2/SOC Estimator (Kalman Filter)1/Kalman Filter/UKF/Correction/updatePk ==
  data: U input; Pk1_k input; Pk1_k1 output; m parameter
function Pk1_k1=updatePk(U,Pk1_k,m)
% Covariance update
%Inputs:
%   U     : U=K*Py'
%   Pk1_k : Covariance at last sample
%   m     : Number of measurements
%Output:
%   Pk1_k1: Updated covariance matrix at (k+1)

% Iterate from 1 to number of measurements

Pk1_k1=battery.control.estimators.CovarianceUpdate(U,Pk1_k,m);

== matlab function EV_Modeling_old/LV/SOC Estimator (Kalman Filter)/Kalman Filter/UKF/Correction/updatePk ==
  data: U input; Pk1_k input; Pk1_k1 output; m parameter
function Pk1_k1=updatePk(U,Pk1_k,m)
% Covariance update
%Inputs:
%   U     : U=K*Py'
%   Pk1_k : Covariance at last sample
%   m     : Number of measurements
%Output:
%   Pk1_k1: Updated covariance matrix at (k+1)

% Iterate from 1 to number of measurements

Pk1_k1=battery.control.estimators.CovarianceUpdate(U,Pk1_k,m);

== matlab function EV_Modeling_old/FV2/SOC Estimator (Kalman Filter)1/Kalman Filter/UKF/Prediction/updatePx ==
  data: X input; x input; Pk1k output; X1 output; Wc parameter; Q parameter
function [Pk1k,X1]=updateP(X,x, Wc, Q)
% Transformed square root of covariance matrix
%Inputs:
%    X  : Sigma points
%    x  : xhat(k+1|k)
%    Wc : Covariance weight 
%    Q  : Covariance of the process noise
%Outputs:
%    Pk1_k: transformed square root of covariance
%    X1: transformed deviations

[Pk1k,X1]=battery.control.estimators.UnscentedTransformationUpdate(X,x, Wc, Q);

== matlab function EV_Modeling_old/FV2/SOC Estimator (Kalman Filter)1/Kalman Filter/UKF/Prediction/updatePy ==
  data: Y input; y input; Py output; Y1 output; Wc parameter; R parameter
function [Py,Y1]=updatePy(Y,y, Wc, R)
% Transformed square root of covariance matrix
%Inputs:
%    Y  : Sigma points
%    y  : yhat(k+1|k)
%    Wc : Covariance weight 
%    R  : Covariance of the measurement noise
%Outputs:
%    Py: transformed square root of covariance
%    Y1: transformed deviations

[Py,Y1]=battery.control.estimators.UnscentedTransformationUpdate(Y,y, Wc, R);

== matlab function EV_Modeling_old/FV2/SOC Estimator (Kalman Filter)1/Kalman Filter/UKF 2RC/Correction/updatePk ==
  data: U input; Pk1_k input; Pk1_k1 output; m parameter
function Pk1_k1=updatePk(U,Pk1_k,m)
% Covariance update
%Inputs:
%   U     : U=K*Py'
%   Pk1_k : Covariance at last sample
%   m     : Number of measurements
%Output:
%   Pk1_k1: Updated covariance matrix at (k+1)

% Iterate from 1 to number of measurements

Pk1_k1=battery.control.estimators.CovarianceUpdate(U,Pk1_k,m);

== matlab function EV_Modeling_old/FV2/SOC Estimator (Kalman Filter)1/Kalman Filter/UKF 2RC/Prediction/updatePx ==
  data: X input; x input; Pk1k output; X1 output; Wc parameter; Q_2RC parameter
function [Pk1k,X1]=updateP(X,x, Wc, Q_2RC)
% Transformed square root of covariance matrix
%Inputs:
%    X  : Sigma points
%    x  : xhat(k+1|k)
%    Wc : Covariance weight 
%    Q  : Covariance of the process noise
%Outputs:
%    Pk1_k: transformed square root of covariance
%    X1: transformed deviations

[Pk1k,X1]=battery.control.estimators.UnscentedTransformationUpdate(X,x, Wc, Q_2RC);

== matlab function EV_Modeling_old/FV1/ACC system/MATLAB Function ==
  data: accel input; acceleration output
function acceleration  = fcn(accel)

if accel > 0 
    acceleration = (accel * 100)/0.15;
elseif accel < 0 
    acceleration = (accel * 100)/0.33;
else
    acceleration = 0; % accel이 0이거나 NaN일 경우에도 대응
end

== matlab function EV_Modeling_old/FV2/SOC Estimator (Kalman Filter)1/Kalman Filter/UKF 2RC/Prediction/updatePy ==
  data: Y input; y input; Py output; Y1 output; Wc parameter; R parameter
function [Py,Y1]=updatePy(Y,y, Wc, R)
% Transformed square root of covariance matrix
%Inputs:
%    Y  : Sigma points
%    y  : yhat(k+1|k)
%    Wc : Covariance weight 
%    R  : Covariance of the measurement noise
%Outputs:
%    Py: transformed square root of covariance
%    Y1: transformed deviations

[Py,Y1]=battery.control.estimators.UnscentedTransformationUpdate(Y,y, Wc, R);

== matlab function EV_Modeling_old/LV/SOC Estimator (Kalman Filter)/Kalman Filter/UKF/Prediction/updatePx ==
  data: X input; x input; Pk1k output; X1 output; Wc parameter; Q parameter
function [Pk1k,X1]=updateP(X,x, Wc, Q)
% Transformed square root of covariance matrix
%Inputs:
%    X  : Sigma points
%    x  : xhat(k+1|k)
%    Wc : Covariance weight 
%    Q  : Covariance of the process noise
%Outputs:
%    Pk1_k: transformed square root of covariance
%    X1: transformed deviations

[Pk1k,X1]=battery.control.estimators.UnscentedTransformationUpdate(X,x, Wc, Q);

== matlab function EV_Modeling_old/LV/SOC Estimator (Kalman Filter)/Kalman Filter/UKF/Prediction/updatePy ==
  data: Y input; y input; Py output; Y1 output; Wc parameter; R parameter
function [Py,Y1]=updatePy(Y,y, Wc, R)
% Transformed square root of covariance matrix
%Inputs:
%    Y  : Sigma points
%    y  : yhat(k+1|k)
%    Wc : Covariance weight 
%    R  : Covariance of the measurement noise
%Outputs:
%    Py: transformed square root of covariance
%    Y1: transformed deviations

[Py,Y1]=battery.control.estimators.UnscentedTransformationUpdate(Y,y, Wc, R);

== matlab function EV_Modeling_old/LV/SOC Estimator (Kalman Filter)/Kalman Filter/UKF 2RC/Correction/updatePk ==
  data: U input; Pk1_k input; Pk1_k1 output; m parameter
function Pk1_k1=updatePk(U,Pk1_k,m)
% Covariance update
%Inputs:
%   U     : U=K*Py'
%   Pk1_k : Covariance at last sample
%   m     : Number of measurements
%Output:
%   Pk1_k1: Updated covariance matrix at (k+1)

% Iterate from 1 to number of measurements

Pk1_k1=battery.control.estimators.CovarianceUpdate(U,Pk1_k,m);

== matlab function EV_Modeling_old/LV/SOC Estimator (Kalman Filter)/Kalman Filter/UKF 2RC/Prediction/updatePx ==
  data: X input; x input; Pk1k output; X1 output; Wc parameter; Q_2RC parameter
function [Pk1k,X1]=updateP(X,x, Wc, Q_2RC)
% Transformed square root of covariance matrix
%Inputs:
%    X  : Sigma points
%    x  : xhat(k+1|k)
%    Wc : Covariance weight 
%    Q  : Covariance of the process noise
%Outputs:
%    Pk1_k: transformed square root of covariance
%    X1: transformed deviations

[Pk1k,X1]=battery.control.estimators.UnscentedTransformationUpdate(X,x, Wc, Q_2RC);

== matlab function EV_Modeling_old/LV/SOC Estimator (Kalman Filter)/Kalman Filter/UKF 2RC/Prediction/updatePy ==
  data: Y input; y input; Py output; Y1 output; Wc parameter; R parameter
function [Py,Y1]=updatePy(Y,y, Wc, R)
% Transformed square root of covariance matrix
%Inputs:
%    Y  : Sigma points
%    y  : yhat(k+1|k)
%    Wc : Covariance weight 
%    R  : Covariance of the measurement noise
%Outputs:
%    Py: transformed square root of covariance
%    Y1: transformed deviations

[Py,Y1]=battery.control.estimators.UnscentedTransformationUpdate(Y,y, Wc, R);

== matlab function EV_Modeling_old/FV1/MATLAB Function ==
  data: Pmotor input; Vbatt input; R output
function R = calcResistance(Pmotor, Vbatt)
    if Pmotor == 0
        R = 1e6; % 매우 큰 저항값으로 설정 (무부하 상태 가정)
    else
        R = (Vbatt^2) / Pmotor;
    end
end

== matlab function EV_Modeling_old/LV/MATLAB Function ==
  data: Pmotor input; Vbatt input; R output
function R = calcResistance(Pmotor, Vbatt)
    if Pmotor == 0
        R = 1e6; % 매우 큰 저항값으로 설정 (무부하 상태 가정)
    else
        R = (Vbatt^2) / Pmotor;
    end
end

== matlab function EV_Modeling_old/FV1/SOC Estimator (Kalman Filter)1/Kalman Filter/UKF/Correction/updatePk ==
  data: U input; Pk1_k input; Pk1_k1 output; m parameter
function Pk1_k1=updatePk(U,Pk1_k,m)
% Covariance update
%Inputs:
%   U     : U=K*Py'
%   Pk1_k : Covariance at last sample
%   m     : Number of measurements
%Output:
%   Pk1_k1: Updated covariance matrix at (k+1)

% Iterate from 1 to number of measurements

Pk1_k1=battery.control.estimators.CovarianceUpdate(U,Pk1_k,m);

== matlab function EV_Modeling_old/FV1/SOC Estimator (Kalman Filter)1/Kalman Filter/UKF/Prediction/updatePx ==
  data: X input; x input; Pk1k output; X1 output; Wc parameter; Q parameter
function [Pk1k,X1]=updateP(X,x, Wc, Q)
% Transformed square root of covariance matrix
%Inputs:
%    X  : Sigma points
%    x  : xhat(k+1|k)
%    Wc : Covariance weight 
%    Q  : Covariance of the process noise
%Outputs:
%    Pk1_k: transformed square root of covariance
%    X1: transformed deviations

[Pk1k,X1]=battery.control.estimators.UnscentedTransformationUpdate(X,x, Wc, Q);

== matlab function EV_Modeling_old/FV1/SOC Estimator (Kalman Filter)1/Kalman Filter/UKF/Prediction/updatePy ==
  data: Y input; y input; Py output; Y1 output; Wc parameter; R parameter
function [Py,Y1]=updatePy(Y,y, Wc, R)
% Transformed square root of covariance matrix
%Inputs:
%    Y  : Sigma points
%    y  : yhat(k+1|k)
%    Wc : Covariance weight 
%    R  : Covariance of the measurement noise
%Outputs:
%    Py: transformed square root of covariance
%    Y1: transformed deviations

[Py,Y1]=battery.control.estimators.UnscentedTransformationUpdate(Y,y, Wc, R);

== matlab function EV_Modeling_old/FV1/SOC Estimator (Kalman Filter)1/Kalman Filter/UKF 2RC/Correction/updatePk ==
  data: U input; Pk1_k input; Pk1_k1 output; m parameter
function Pk1_k1=updatePk(U,Pk1_k,m)
% Covariance update
%Inputs:
%   U     : U=K*Py'
%   Pk1_k : Covariance at last sample
%   m     : Number of measurements
%Output:
%   Pk1_k1: Updated covariance matrix at (k+1)

% Iterate from 1 to number of measurements

Pk1_k1=battery.control.estimators.CovarianceUpdate(U,Pk1_k,m);

== matlab function EV_Modeling_old/FV1/SOC Estimator (Kalman Filter)1/Kalman Filter/UKF 2RC/Prediction/updatePx ==
  data: X input; x input; Pk1k output; X1 output; Wc parameter; Q_2RC parameter
function [Pk1k,X1]=updateP(X,x, Wc, Q_2RC)
% Transformed square root of covariance matrix
%Inputs:
%    X  : Sigma points
%    x  : xhat(k+1|k)
%    Wc : Covariance weight 
%    Q  : Covariance of the process noise
%Outputs:
%    Pk1_k: transformed square root of covariance
%    X1: transformed deviations

[Pk1k,X1]=battery.control.estimators.UnscentedTransformationUpdate(X,x, Wc, Q_2RC);
